simulink model "test"  (R2016a)
settings: Solver=VariableStepAuto  StartTime=0.0  StopTime=10.0  RelTol=1e-3
libraries: simulink x1
settings Model: Creator=Administrator  LastModifiedBy=Administrator

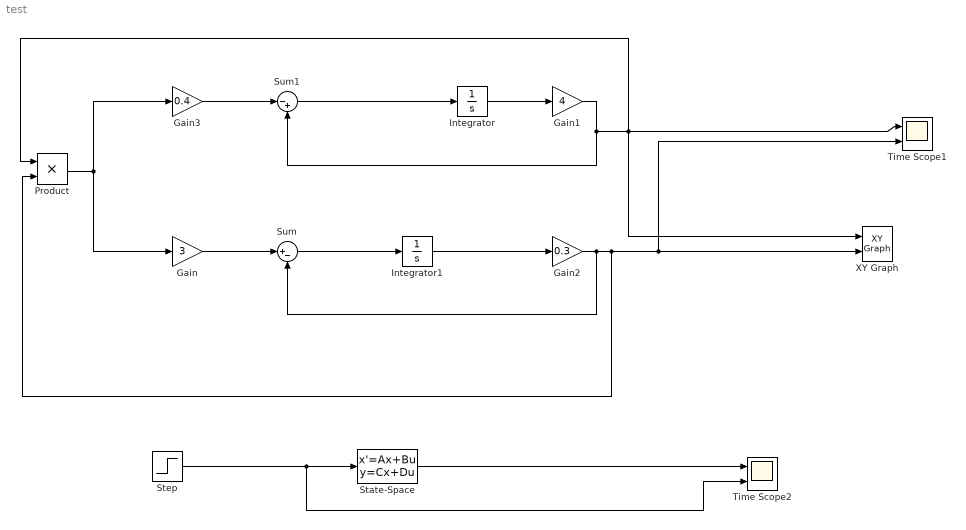
== system test ==
  Gain : Gain  Gain=3
  Gain1 : Gain  Gain=4
  Gain2 : Gain  Gain=0.3
  Gain3 : Gain  Gain=0.4
  Integrator : Integrator
  Integrator1 : Integrator
  Product : Product
  State-Space : StateSpace  A=[0 -0.04; 0.3 0]  B=[1; 0]  C=[1 0]  D=0  X0=0
  Step : Step  Time=0  After=0  SampleTime=0
  Sum : Sum  Inputs=|+-
  Sum1 : Sum  Inputs=|-+
  Time Scope1 : Scope  NumInputPorts=2
  Time Scope2 : Scope  NumInputPorts=2
  XY Graph : simulink/Sinks/XY Graph  xmin=-1  xmax=1  ymin=-1  ymax=1  st=-1
  wires:
  Gain/1 -> Sum/1
  Product/1 -> Gain/1, Gain3/1
  Gain3/1 -> Sum1/1
  Sum1/1 -> Integrator/1
  Sum/1 -> Integrator1/1
  Integrator/1 -> Gain1/1
  Integrator1/1 -> Gain2/1
  Gain1/1 -> XY Graph/1, Time Scope1/1, Product/1, Sum1/2
  Gain2/1 -> Sum/2, Product/2, Time Scope1/2, XY Graph/2
  State-Space/1 -> Time Scope2/1
  Step/1 -> Time Scope2/2, State-Space/1
